simulink model "MPC_Simulator"  (R2024a)
settings: Solver=VariableStepAuto  StartTime=0.0  StopTime=20  RelTol=1e-3
values from neighbouring files (symbols this model uses):
  A_Matrix_QP_Cons = [-1 0 0;1 0 0]    [MPC_Implementation_Tests.m]
  b_Matrix_QP_Cons = [-2*(pi/180)*T_s;2*(pi/180)*T_s]    [MPC_Implementation_Tests.m]
  C_Ship_Discrete = [1 0]    [MPC_Implementation_Tests.m]
  Gamma = [0;T_s*(K/T)]    [MPC_Implementation_Tests.m]
  Phi = [1 T_s;0 1-(T_s/T)]    [MPC_Implementation_Tests.m]
  Q = eye(3)    [MPC_Implementation_Tests.m]
  R = 0.01*eye(3)    [MPC_Implementation_Tests.m]
  T_s = 0.1    [MPC_Implementation_Tests.m]
  W = [C_Aug*Phi_Aug;C_Aug*Phi_Aug^2;C_Aug*Phi_Aug^N_p]    [MPC_Implementation_Tests.m]
  Z = [C_Aug*Gamma_Aug 0 0;C_Aug*Phi_Aug*Gamma_Aug C_Aug*Gamma_Aug 0;     C_Aug*Phi_Aug^(N_p-1)*Gamma_Aug C_Aug*Phi_Aug*Gamma_Aug C_Aug*Gamma_Aug]    [MPC_Implementation_Tests.m]
undefined symbols (not defined in the file or in its folder): DiscIntNeverNeededParam
settings Model: Creator=gerar  LastModifiedBy=gerar

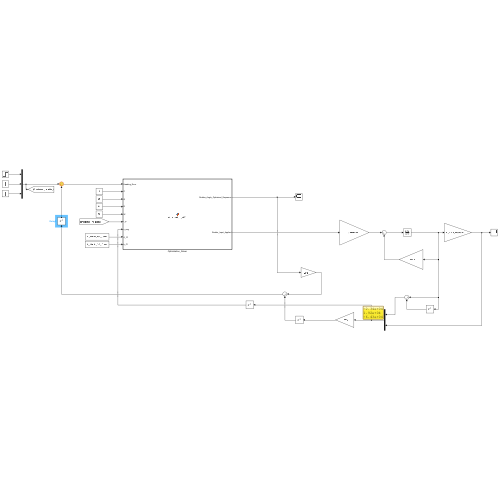
[thumbnail: Simulink's stored preview of the top-level diagram]
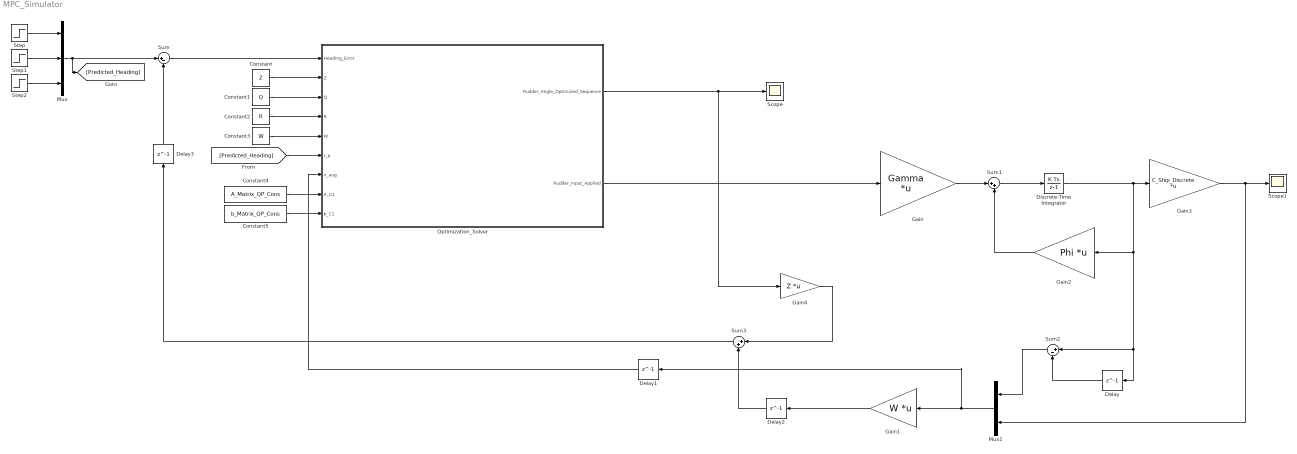
== system MPC_Simulator ==
  Constant : Constant  Value=Z
  Constant1 : Constant  Value=Q
  Constant2 : Constant  Value=R
  Constant3 : Constant  Value=W
  Constant4 : Constant  Value=A_Matrix_QP_Cons
  Constant5 : Constant  Value=b_Matrix_QP_Cons
  Delay : Delay  DelayLength=1  InputProcessing=Columns as channels (frame based)
  Delay1 : Delay  DelayLength=1  InputProcessing=Columns as channels (frame based)  SampleTime=T_s
  Delay2 : Delay  DelayLength=1  InputProcessing=Columns as channels (frame based)  SampleTime=T_s
  Delay3 : Delay  DelayLength=1  InputProcessing=Columns as channels (frame based)  SampleTime=T_s
  Discrete-Time Integrator : DiscreteIntegrator  InitialCondition=[0;0]  SampleTime=T_s  ICPrevOutput=DiscIntNeverNeededParam  ICPrevScaledInput=DiscIntNeverNeededParam
  Gain : Gain  Gain=Gamma  Multiplication=Matrix(K*u)
  Gain1 : Gain  Gain=W  Multiplication=Matrix(K*u)
  Gain2 : Gain  Gain=Phi  Multiplication=Matrix(K*u)
  Gain3 : Gain  Gain=C_Ship_Discrete  Multiplication=Matrix(K*u)
  Gain4 : Gain  Gain=Z  Multiplication=Matrix(K*u)
  Mux : Mux  Inputs=3
  Mux1 : Mux  Inputs=2
  Optimization_Solver : MATLAB Function  TreatAsAtomicUnit=on  SystemSampleTime=T_s
  Scope : Scope
  Scope1 : Scope
  Step : Step  Time=0  After=15*(pi/180)  SampleTime=0
  Step1 : Step  Time=0  After=15*(pi/180)  SampleTime=0
  Step2 : Step  Time=0  After=15*(pi/180)  SampleTime=0
  Sum : Sum  Inputs=|+-
  Sum1 : Sum  Inputs=|++
  Sum2 : Sum  Inputs=|+-
  Sum3 : Sum  Inputs=|++
  wires:
  Step2/1 -> Mux/3
  Step1/1 -> Mux/2
  Step/1 -> Mux/1
  Mux/1 -> [Predicted_Heading], Sum/1
  Sum/1 -> Optimization_Solver/1(Heading_Error)
  Constant/1 -> Optimization_Solver/2(Z)
  Constant1/1 -> Optimization_Solver/3(Q)
  Constant2/1 -> Optimization_Solver/4(R)
  Constant3/1 -> Optimization_Solver/5(W)
  [Predicted_Heading] -> Optimization_Solver/6(r_p)
  Constant4/1 -> Optimization_Solver/8(A_C1)
  Constant5/1 -> Optimization_Solver/9(b_C1)
  Optimization_Solver/2(Rudder_Input_Applied) -> Gain/1
  Gain/1 -> Sum1/1
  Sum1/1 -> Discrete-Time Integrator/1
  Gain2/1 -> Sum1/2
  Discrete-Time Integrator/1 -> Sum2/1, Delay/1, Gain2/1, Gain3/1
  Gain3/1 -> Mux1/2, Scope1/1
  Delay/1 -> Sum2/2
  Sum2/1 -> Mux1/1
  Mux1/1 -> Delay1/1, Gain1/1
  Gain4/1 -> Sum3/1
  Gain1/1 -> Delay2/1
  Delay1/1 -> Optimization_Solver/7(x_aug)
  Sum3/1 -> Delay3/1
  Optimization_Solver/1(Rudder_Angle_Optimized_Sequence) -> Gain4/1, Scope/1
  Delay2/1 -> Sum3/2
  Delay3/1 -> Sum/2

== matlab function MPC_Simulator/Optimization_Solver ==
  data: Heading_Error input; Rudder_Angle_Optimized_Sequence output; Z input; Q input; R input; W input; r_p input; x_aug input; A_C1 input; b_C1 input; Rudder_Input_Applied output
function [Rudder_Angle_Optimized_Sequence,Rudder_Input_Applied] = Optimization_MPC(Heading_Error,...
                                                            Z,...
                                                            Q,...
                                                            R,...
                                                            W,...
                                                            r_p,...
                                                            x_aug,...
                                                            A_C1,...
                                                            b_C1)

% Call to the Matlab function:
[Rudder_Angle_Optimized_Sequence,Rudder_Input_Applied] = EMF_Optimization_MPC(Heading_Error,...
                                                        Z,...
                                                        Q,...
                                                        R,...
                                                        W,...
                                                        r_p,...
                                                        x_aug,...
                                                        A_C1,...
                                                        b_C1);

end
